simulink model "blockdemo"  (Simulink 6.3)
settings: Solver=FixedStepDiscrete  StartTime=0.0  StopTime=200  FixedStep=1  RelTol=1e-3
InitFcn:
  | %% DSPBuilder Start
  | alt_dspbuilder_update_model(bdroot)
  | %% DSPBuilder End
libraries: simulink x1, simulationonly_alteradspbuilder2 x1
settings Model: LastModifiedBy=ggriffit

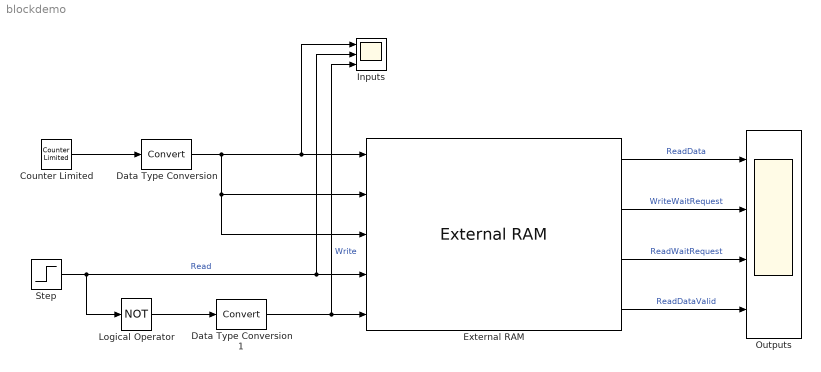
== system blockdemo ==
  Counter Limited : simulink/Sources/Counter Limited  uplimit=100  tsamp=-1
  Data Type Conversion : DataTypeConversion
  Data Type Conversion1 : DataTypeConversion
  External RAM : simulationonly_alteradspbuilder2/External RAM  DATA_WIDTH=32  ADDRESS_WIDTH=8  WAIT_STATES_PER_WRITE=0  MAXIMUM_LATENCY=1  SIZE=200  OFFSET=0
  Inputs : Scope  NumInputPorts=3
      settings: YMin=0~-5~-5  YMax=100~5~5  SampleInput=on
  Logical Operator : Logic  Operator=NOT  AllPortsSameDT=off  OutDataTypeMode=Boolean
  Outputs : Scope  NumInputPorts=4
      settings: YMin=0~-5~-5~-5  YMax=100~5~5~5  SampleInput=on
  Step : Step  Time=100  SampleTime=0
  wires:
  Data Type Conversion/1 -> External RAM/3, External RAM/2, Inputs/1, External RAM/1
  Counter Limited/1 -> Data Type Conversion/1
  Step/1 -> Logical Operator/1, Inputs/2, External RAM/4  "Read"
  Logical Operator/1 -> Data Type Conversion1/1
  Data Type Conversion1/1 -> Inputs/3, External RAM/5  "Write"
  External RAM/1 -> Outputs/1  "ReadData"
  External RAM/2 -> Outputs/2  "WriteWaitRequest"
  External RAM/3 -> Outputs/3  "ReadWaitRequest"
  External RAM/4 -> Outputs/4  "ReadDataValid"
